simulink model "Model_6DOF"  (R2022b)
settings: Solver=VariableStepAuto  StartTime=0.0  StopTime=SimTime  RelTol=1e-6
InitFcn:
  | INIT_DATA
values from neighbouring files (symbols this model uses):
  g = 9.81    [aero_guid_dat.m]
  K_r = -0.02    [aero_guid_dat.m]
undefined symbols (not defined in the file or in its folder): a_L_c_max, a_N_c_max, b, C_bar, C_D_0, C_D_0_bar, C_D_alpha, C_D_d_e, C_L_0, C_L_0_bar, C_L_alpha, C_l_beta, C_l_d_a, C_L_d_e, C_l_d_r, C_l_p, C_L_q, C_l_r, C_m_0, C_m_alpha, C_m_d_e, C_m_q, C_n_beta, C_n_d_a, C_n_d_r, C_n_p, C_n_r, C_y_beta, C_y_d_a, C_y_d_r, C_y_p, C_y_r, d_T, da_max, da_rate_max, de_max, de_rate_max, dr_max, dr_rate_max, E, EA0, eR_0_IhI_Ih, eS_0_BE_Lh, eV_0_BE_Lh, G_cp, G_I, G_M, G_M_I, G_R, G_s, GC, I, INS_bias_f, INS_bias_omega, INS_imbalance_error, INS_scale_factor_error_f, INS_scale_factor_error_omega, k, K_beta, K_p ... (+34)
libraries: dspsrcs4 x11, matrix_library x6, simulink x5, sharedutil x3, aerolibasang x3, sharedtransform x2, simulink_extras x1, slpidlib x1
(part 1 of 2)
settings Model: Creator=Milad  LastModifiedBy=Mahdi
settings SolverCC: AlgebraicLoopSolver=TrustRegion
settings OptimizationCC: LifeSpan=inf
settings DebuggingCC: UnconnectedInputMsg=warning  UnconnectedOutputMsg=warning  UnconnectedLineMsg=warning  SFExecutionAtInitializationDiag=none  SFMachineParentedDataDiag=warning  ArithmeticOperatorsInVariantConditions=warning
settings HardwareCC: ProdBitPerSizeT=32  ProdBitPerPtrDiffT=32  ProdWordSize=32  ProdHWDeviceType=Specified
settings ModelReferenceCC: EnableRefExpFcnMdlSchedulingChecks=on
settings SFSimCC: CustomCodeUndefinedFunction=UseInterfaceOnly
settings CodeAppCC: StateflowObjectComments=on

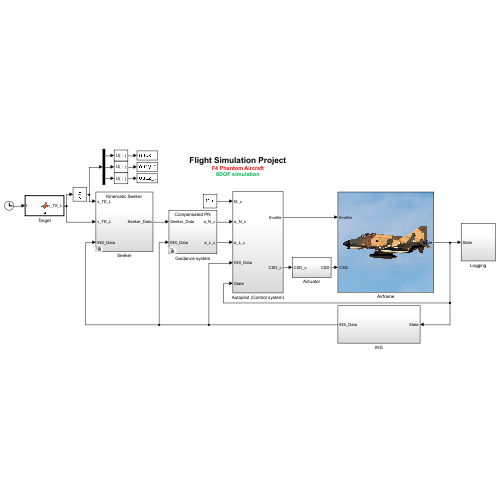
[thumbnail: Simulink's stored preview of the top-level diagram]
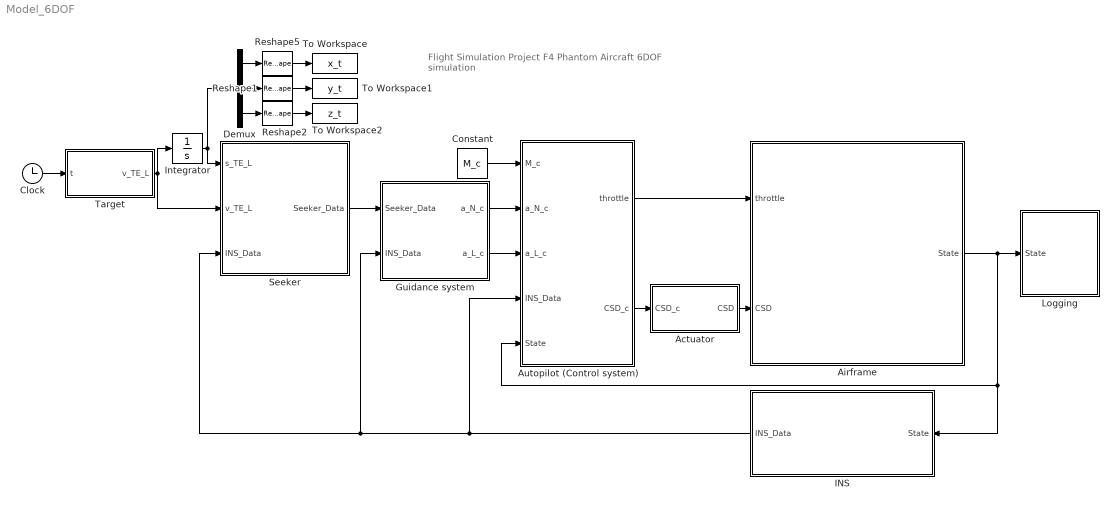
== system Model_6DOF ==
  note: Flight Simulation Project
      | F4 Phantom Aircraft
      | 6DOF simulation
  Actuator : Subsystem
  Airframe : Subsystem
      mask Display: image('E:\term courses\FS\project\phase1\70285_1544476732.jpg'); % Use "Edit Image" on toolstrip to change.
  Autopilot (Control system) : Subsystem
  Clock : Clock
  Constant : Constant  Value=M_c
  Demux : Demux  Outputs=3
  Guidance system : Subsystem  Variant=on  VariantControlMode=label  VariantControl=Choice  LabelModeActiveChoice=CPN
  INS : Subsystem
  Integrator : Integrator  InitialCondition=s_TE_L_0
  Logging : Subsystem
  Reshape1 : Reshape
  Reshape2 : Reshape
  Reshape5 : Reshape
  Seeker : Subsystem  Variant=on  VariantControlMode=label  VariantControl=Choice  LabelModeActiveChoice=kinematic
  Target : MATLAB Function  TreatAsAtomicUnit=on
  To Workspace : ToWorkspace  VariableName=x_t  SampleTime=out_SampleTime
  To Workspace1 : ToWorkspace  VariableName=y_t  SampleTime=out_SampleTime
  To Workspace2 : ToWorkspace  VariableName=z_t  SampleTime=out_SampleTime
  wires:
  Airframe/1(State) -> Logging/1(State), INS/1(State), Autopilot (Control system)/5(State)
  Autopilot (Control system)/1(throttle) -> Airframe/1(throttle)
  Autopilot (Control system)/2(CSD_c) -> Actuator/1(CSD_c)
  INS/1(INS_Data) -> Seeker/3(INS_Data), Guidance system/2(INS_Data), Autopilot (Control system)/4(INS_Data)
  Clock/1 -> Target/1(t)
  Reshape1/1 -> To Workspace1/1
  Reshape2/1 -> To Workspace2/1
  Demux/2 -> Reshape1/1
  Integrator/1 -> Demux/1, Seeker/1(s_TE_L)
  Target/1(v_TE_L) -> Seeker/2(v_TE_L), Integrator/1
  Demux/3 -> Reshape2/1
  Constant/1 -> Autopilot (Control system)/1(M_c)
  Demux/1 -> Reshape5/1
  Reshape5/1 -> To Workspace/1
  Actuator/1(CSD) -> Airframe/2(CSD)
  Guidance system/1(a_N_c) -> Autopilot (Control system)/2(a_N_c)
  Guidance system/2(a_L_c) -> Autopilot (Control system)/3(a_L_c)
  Seeker/1(Seeker_Data) -> Guidance system/1(Seeker_Data)

== system Model_6DOF/Actuator ==
  CSD_c : Inport
  Aileron Actuator Transfer Function : Subsystem
  Demux : Demux  Outputs=3
  Elevator Actuator Transfer Function : Subsystem
  Mux : Mux  Inputs=3
  Rudder Actuator Transfer Function : Subsystem
  CSD : Outport
  wires:
  Elevator Actuator Transfer Function/1(de) -> Mux/1
  Mux/1 -> CSD/1
  CSD_c/1 -> Demux/1
  Demux/1 -> Elevator Actuator Transfer Function/1(de_c)
  Demux/2 -> Aileron Actuator Transfer Function/1(da_c)
  Aileron Actuator Transfer Function/1(da) -> Mux/2
  Demux/3 -> Rudder Actuator Transfer Function/1(dr_c)
  Rudder Actuator Transfer Function/1(dr) -> Mux/3

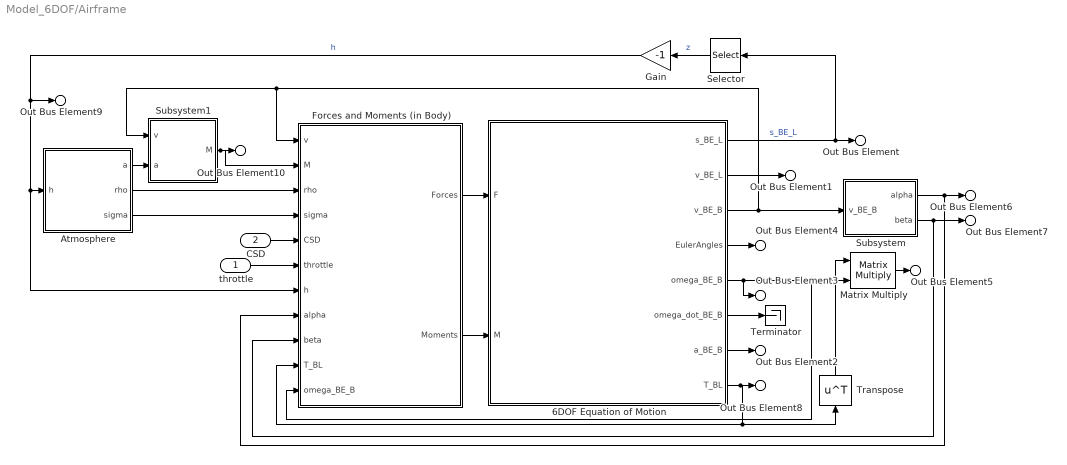
== system Model_6DOF/Airframe ==
  throttle : Inport
  CSD : Inport  Port=2
  6DOF Equation of Motion : Subsystem
  Atmosphere : MATLAB Function  TreatAsAtomicUnit=on
  Forces and Moments (in Body) : Subsystem
  Gain : Gain  Gain=-1
  Matrix Multiply : Product  Multiplication=Matrix(*)
  Selector : Selector  InputPortWidth=3  IndexOptions=Index vector (dialog)  Indices=3  OutputSizes=1
  Subsystem : Subsystem
  Subsystem1 : Subsystem
  Terminator : Terminator
  Transpose : Math  Operator=transpose
  Out Bus Element : Outport  PortName=State  Element=s_BE_L
  Out Bus Element1 : Outport  PortName=State  Element=v_BE_L
  Out Bus Element2 : Outport  PortName=State  Element=f_sp_B
  Out Bus Element3 : Outport  PortName=State  Element=omega_BE_B
  Out Bus Element4 : Outport  PortName=State  Element=EulerAngles
  Out Bus Element5 : Outport  PortName=State  Element=Omega_BE_L
  Out Bus Element6 : Outport  PortName=State  Element=alpha
  Out Bus Element7 : Outport  PortName=State  Element=beta
  Out Bus Element8 : Outport  PortName=State  Element=T_BL
  Out Bus Element9 : Outport  PortName=State  Element=h
  Out Bus Element10 : Outport  PortName=State  Element=M
  wires:
  6DOF Equation of Motion/2(v_BE_L) -> Out Bus Element1/1
  6DOF Equation of Motion/1(s_BE_L) -> Out Bus Element/1, Selector/1  "s_BE_L"
  Selector/1 -> Gain/1  "z"
  Gain/1 -> Out Bus Element9/1, Forces and Moments (in Body)/7(h), Atmosphere/1(h)  "h"
  Atmosphere/2(rho) -> Forces and Moments (in Body)/3(rho)
  Subsystem/1(alpha) -> Out Bus Element6/1, Forces and Moments (in Body)/8(alpha)
  Subsystem/2(beta) -> Out Bus Element7/1, Forces and Moments (in Body)/9(beta)
  throttle/1 -> Forces and Moments (in Body)/6(throttle)
  6DOF Equation of Motion/8(T_BL) -> Transpose/1, Forces and Moments (in Body)/10(T_BL), Out Bus Element8/1
  6DOF Equation of Motion/7(a_BE_B) -> Out Bus Element2/1
  Matrix Multiply/1 -> Out Bus Element5/1
  Atmosphere/3(sigma) -> Forces and Moments (in Body)/4(sigma)
  6DOF Equation of Motion/3(v_BE_B) -> Subsystem1/1(v), Forces and Moments (in Body)/1(v), Subsystem/1(v_BE_B)
  Forces and Moments (in Body)/1(Forces) -> 6DOF Equation of Motion/1(" F")
  Atmosphere/1(a) -> Subsystem1/2(a)
  Subsystem1/1(M) -> Forces and Moments (in Body)/2(M), Out Bus Element10/1
  Forces and Moments (in Body)/2(Moments) -> 6DOF Equation of Motion/2(M)
  CSD/1 -> Forces and Moments (in Body)/5(CSD)
  6DOF Equation of Motion/4(EulerAngles) -> Out Bus Element4/1
  6DOF Equation of Motion/5(omega_BE_B) -> Out Bus Element3/1, Matrix Multiply/2, Forces and Moments (in Body)/11(omega_BE_B)
  Transpose/1 -> Matrix Multiply/1
  6DOF Equation of Motion/6(omega_dot_BE_B) -> Terminator/1

== system Model_6DOF/Autopilot (Control system) ==
  M_c : Inport
  a_N_c : Inport  Port=2
  a_L_c : Inport  Port=3
  INS_Data : Inport  Port=4
  BusElementIn : Inport  Port=5  PortName=State  Element=h
  BusElementIn1 : Inport  Port=5  PortName=State  Element=beta
  BusElementIn2 : Inport  Port=5  PortName=State  Element=alpha
  BusElementIn3 : Inport  Port=5  PortName=State  Element=M
  Acceleration Autopilot : Subsystem
  Mach Hold Autopilot : Subsystem
  Mux : Mux  Inputs=3
  beta control : Subsystem
  throttle : Outport
  CSD_c : Outport  Port=2
  wires:
  M_c/1 -> Mach Hold Autopilot/1(M_c)
  Mach Hold Autopilot/1(throttle) -> throttle/1
  Acceleration Autopilot/1(de_c) -> Mux/1  "de_c"
  a_N_c/1 -> Acceleration Autopilot/1(a_N_c)
  a_L_c/1 -> Acceleration Autopilot/2(a_L_c)
  INS_Data/1 -> beta control/1(INS_Data), Acceleration Autopilot/3(INS_Data)
  Acceleration Autopilot/2(da_c) -> Mux/2  "da_c"
  beta control/1(dr_c) -> Mux/3
  Mux/1 -> CSD_c/1
  BusElementIn1/1 -> beta control/2(beta)
  BusElementIn/1 -> Mach Hold Autopilot/3(h)
  BusElementIn2/1 -> Mach Hold Autopilot/4(alpha)
  BusElementIn3/1 -> Mach Hold Autopilot/2(M)

== system Model_6DOF/Guidance system ==
  Seeker_Data : Inport
  INS_Data : Inport  Port=2
  Compensated PN : Subsystem  VariantControl=CPN
  IPN : Subsystem  VariantControl=IPN
  Optimal Guidance : Subsystem  VariantControl=OG
  a_N_c : Outport
  a_L_c : Outport  Port=2

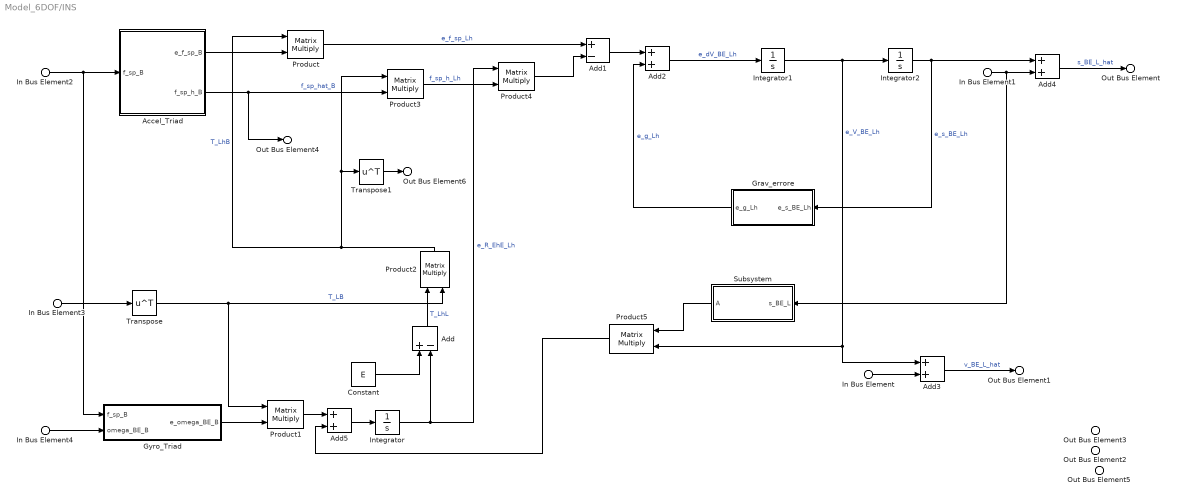
== system Model_6DOF/INS ==
  In Bus Element : Inport  PortName=State  Element=v_BE_L
  In Bus Element1 : Inport  PortName=State  Element=s_BE_L
  In Bus Element2 : Inport  PortName=State  Element=f_sp_B
  In Bus Element3 : Inport  PortName=State  Element=T_BL
  In Bus Element4 : Inport  PortName=State  Element=omega_BE_B
  Accel_Triad : Subsystem
  Add : Sum  Inputs=+-
  Add1 : Sum  Inputs=+-
  Add{2..5} (4 alike) : Sum
  Constant : Constant  Value=E
  Grav_errore : Subsystem
  Gyro_Triad : Subsystem
  Integrator : Integrator  InitialCondition=eR_0_IhI_Ih
  Integrator1 : Integrator  InitialCondition=eV_0_BE_Lh
  Integrator2 : Integrator  InitialCondition=eS_0_BE_Lh
  Product{,1..5} (6 alike) : Product  Multiplication=Matrix(*)
  Subsystem : Subsystem
  Transpose : Math  Operator=transpose
  Transpose1 : Math  Operator=transpose
  Out Bus Element : Outport  PortName=INS_Data  Element=s_BE_L_hat
  Out Bus Element1 : Outport  PortName=INS_Data  Element=v_BE_L_hat
  Out Bus Element2 : Outport  PortName=INS_Data  Element=phi_theta_psi
  Out Bus Element3 : Outport  PortName=INS_Data  Element=pqr
  Out Bus Element4 : Outport  PortName=INS_Data  Element=f_sp_hat_B
  Out Bus Element5 : Outport  PortName=INS_Data  Element=a_m
  Out Bus Element6 : Outport  PortName=INS_Data  Element=T_BL_hat
  wires:
  ? -> Out Bus Element3/1
  ? -> Out Bus Element2/1
  Accel_Triad/2(f_sp_h_B) -> Out Bus Element4/1, Product3/2  "f_sp_hat_B"
  Transpose1/1 -> Out Bus Element6/1
  ? -> Out Bus Element5/1
  In Bus Element/1 -> Add3/2
  Product5/1 -> Add5/2
  Product1/1 -> Add5/1
  Integrator2/1 -> Grav_errore/1(e_s_BE_Lh), Add4/1  "e_s_BE_Lh"
  Integrator1/1 -> Integrator2/1, Product5/2, Add3/1  "e_V_BE_Lh"
  Accel_Triad/1(e_f_sp_B) -> Product/2
  Product3/1 -> Product4/2  "f_sp_h_Lh"
  Gyro_Triad/1(e_omega_BE_B) -> Product1/2
  Add/1 -> Product2/1  "T_LhL"
  Add5/1 -> Integrator/1
  Product/1 -> Add1/1  "e_f_sp_Lh"
  Add2/1 -> Integrator1/1  "e_dV_BE_Lh"
  Constant/1 -> Add/1
  Add4/1 -> Out Bus Element/1  "s_BE_L_hat"
  Add3/1 -> Out Bus Element1/1  "v_BE_L_hat"
  Integrator/1 -> Add/2, Product4/1  "e_R_EhE_Lh"
  Product4/1 -> Add1/2
  Add1/1 -> Add2/1
  Product2/1 -> Product3/1, Transpose1/1, Product/1  "T_LhB"
  Grav_errore/1(e_g_Lh) -> Add2/2  "e_g_Lh"
  Transpose/1 -> Product1/1, Product2/2  "T_LB"
  Subsystem/1(A) -> Product5/1
  In Bus Element1/1 -> Subsystem/1(s_BE_L), Add4/2
  In Bus Element2/1 -> Gyro_Triad/1(f_sp_B), Accel_Triad/1(f_sp_B)
  In Bus Element3/1 -> Transpose/1
  In Bus Element4/1 -> Gyro_Triad/2(omega_BE_B)

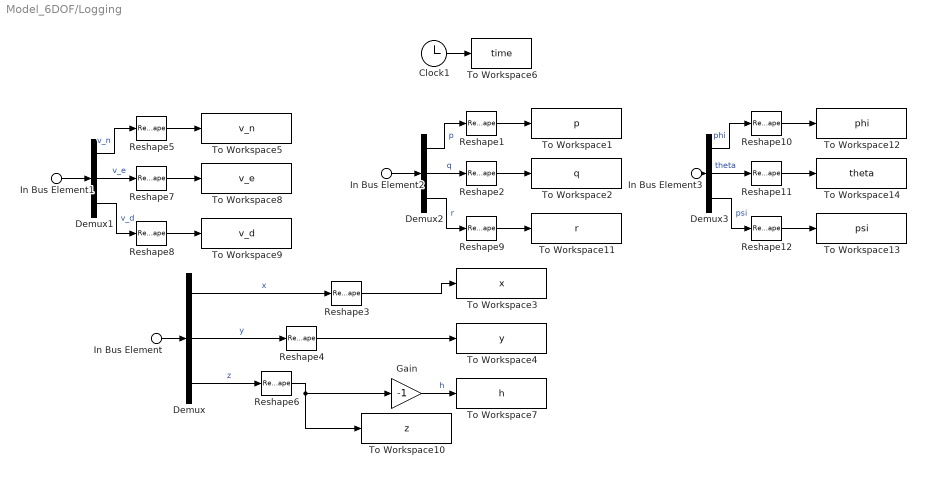
== system Model_6DOF/Logging ==
  In Bus Element : Inport  PortName=State  Element=s_BE_L
  In Bus Element1 : Inport  PortName=State  Element=v_BE_L
  In Bus Element2 : Inport  PortName=State  Element=omega_BE_B
  In Bus Element3 : Inport  PortName=State  Element=EulerAngles
  Clock1 : Clock
  Demux{,1..3} (4 alike) : Demux  Outputs=3
  Gain : Gain  Gain=-1
  Reshape{1..12} (12 alike) : Reshape
  To Workspace1 : ToWorkspace  VariableName=p  SampleTime=out_SampleTime
  To Workspace10 : ToWorkspace  VariableName=z  SampleTime=out_SampleTime
  To Workspace11 : ToWorkspace  VariableName=r  SampleTime=out_SampleTime
  To Workspace12 : ToWorkspace  VariableName=phi  SampleTime=out_SampleTime
  To Workspace13 : ToWorkspace  VariableName=psi  SampleTime=out_SampleTime
  To Workspace14 : ToWorkspace  VariableName=theta  SampleTime=out_SampleTime
  To Workspace2 : ToWorkspace  VariableName=q  SampleTime=out_SampleTime
  To Workspace3 : ToWorkspace  VariableName=x  SampleTime=out_SampleTime
  To Workspace4 : ToWorkspace  VariableName=y  SampleTime=out_SampleTime
  To Workspace5 : ToWorkspace  VariableName=v_n  SampleTime=out_SampleTime
  To Workspace6 : ToWorkspace  VariableName=time  SampleTime=out_SampleTime
  To Workspace7 : ToWorkspace  VariableName=h  SampleTime=out_SampleTime
  To Workspace8 : ToWorkspace  VariableName=v_e  SampleTime=out_SampleTime
  To Workspace9 : ToWorkspace  VariableName=v_d  SampleTime=out_SampleTime
  wires:
  Clock1/1 -> To Workspace6/1
  Demux/3 -> Reshape6/1  "z"
  Demux/1 -> Reshape3/1  "x"
  Gain/1 -> To Workspace7/1  "h"
  Demux/2 -> Reshape4/1  "y"
  In Bus Element1/1 -> Demux1/1
  Demux1/1 -> Reshape5/1  "v_n"
  Demux1/2 -> Reshape7/1  "v_e"
  Demux1/3 -> Reshape8/1  "v_d"
  Reshape3/1 -> To Workspace3/1
  Reshape4/1 -> To Workspace4/1
  Reshape6/1 -> Gain/1, To Workspace10/1
  Reshape5/1 -> To Workspace5/1
  Reshape7/1 -> To Workspace8/1
  Reshape8/1 -> To Workspace9/1
  In Bus Element/1 -> Demux/1
  In Bus Element2/1 -> Demux2/1
  Demux2/3 -> Reshape9/1  "r"
  Reshape9/1 -> To Workspace11/1
  Reshape2/1 -> To Workspace2/1
  Demux2/2 -> Reshape2/1  "q"
  Demux2/1 -> Reshape1/1  "p"
  Reshape1/1 -> To Workspace1/1
  Reshape10/1 -> To Workspace12/1
  Demux3/1 -> Reshape10/1  "phi"
  Demux3/2 -> Reshape11/1  "theta"
  Reshape11/1 -> To Workspace14/1
  Demux3/3 -> Reshape12/1  "psi"
  In Bus Element3/1 -> Demux3/1
  Reshape12/1 -> To Workspace13/1

== system Model_6DOF/Seeker ==
  s_TE_L : Inport
  v_TE_L : Inport  Port=2
  INS_Data : Inport  Port=3
  Dynamic Seeker : Subsystem  VariantControl=dynamic
  Kinematic Seeker : Subsystem  VariantControl=kinematic
  Seeker_Data : Outport

== system Model_6DOF/Actuator/Aileron Actuator Transfer Function ==
  da_c : Inport
  Gain : Gain  Gain=omega_n_da^2
  Gain1 : Gain  Gain=2*zeta_da
  Gain2 : Gain  Gain=omega_n_da
  Integrator : Integrator
  Integrator1 : Integrator
  Rate Saturation : Saturate  UpperLimit=da_rate_max  LowerLimit=-da_rate_max
  Sum : Sum  Inputs=|+-
  Sum1 : Sum  Inputs=|+-
  deflection saturation : Saturate  UpperLimit=da_max  LowerLimit=-da_max
  da : Outport
  wires:
  deflection saturation/1 -> da/1, Sum/2
  Integrator1/1 -> deflection saturation/1
  Rate Saturation/1 -> Gain1/1, Integrator1/1
  Integrator/1 -> Rate Saturation/1
  Sum1/1 -> Integrator/1
  Gain2/1 -> Sum1/2
  Gain1/1 -> Gain2/1
  Gain/1 -> Sum1/1
  Sum/1 -> Gain/1
  da_c/1 -> Sum/1

== system Model_6DOF/Actuator/Elevator Actuator Transfer Function ==
  de_c : Inport
  Gain : Gain  Gain=omega_n_de^2
  Gain1 : Gain  Gain=2*zeta_de
  Gain2 : Gain  Gain=omega_n_de
  Integrator : Integrator
  Integrator1 : Integrator
  Rate Saturation : Saturate  UpperLimit=de_rate_max  LowerLimit=-de_rate_max
  Sum : Sum  Inputs=|+-
  Sum1 : Sum  Inputs=|+-
  deflection saturation : Saturate  UpperLimit=de_max  LowerLimit=-de_max
  de : Outport
  wires:
  de_c/1 -> Sum/1
  Sum/1 -> Gain/1
  Gain/1 -> Sum1/1
  Gain1/1 -> Gain2/1
  Gain2/1 -> Sum1/2
  Sum1/1 -> Integrator/1
  Integrator/1 -> Rate Saturation/1
  Rate Saturation/1 -> Integrator1/1, Gain1/1
  Integrator1/1 -> deflection saturation/1
  deflection saturation/1 -> Sum/2, de/1

== system Model_6DOF/Actuator/Rudder Actuator Transfer Function ==
  dr_c : Inport
  Gain : Gain  Gain=omega_n_dr^2
  Gain1 : Gain  Gain=2*zeta_dr
  Gain2 : Gain  Gain=omega_n_dr
  Integrator : Integrator
  Integrator1 : Integrator
  Rate Saturation : Saturate  UpperLimit=dr_rate_max  LowerLimit=-dr_rate_max
  Sum : Sum  Inputs=|+-
  Sum1 : Sum  Inputs=|+-
  deflection saturation : Saturate  UpperLimit=dr_max  LowerLimit=-dr_max
  dr : Outport
  wires:
  dr_c/1 -> Sum/1
  Sum/1 -> Gain/1
  Gain/1 -> Sum1/1
  Gain1/1 -> Gain2/1
  Gain2/1 -> Sum1/2
  Sum1/1 -> Integrator/1
  Integrator/1 -> Rate Saturation/1
  Rate Saturation/1 -> Integrator1/1, Gain1/1
  Integrator1/1 -> deflection saturation/1
  deflection saturation/1 -> Sum/2, dr/1

== system Model_6DOF/Airframe/6DOF Equation of Motion ==
  " F" : Inport
  M : Inport  Port=2
  Demux : Demux  Outputs=3
  Integrator : Integrator  InitialCondition=Vb0
  Integrator1 : Integrator  InitialCondition=X0
  Integrator2 : Integrator  InitialCondition=RR0
  Integrator3 : Integrator  InitialCondition=EA0  WrapState=on
  Mux : Mux  Inputs=3
  Rotation Angles to Direction Cosine Matrix : sharedtransform/Rotation Angles to Direction Cosine Matrix  rotationOrder=ZYX  aMode=aMode
  Rotational Dynamics (kinetics) : Subsystem
  Rotational Kinematics : Subsystem
  Saturation : Saturate  UpperLimit=0  LowerLimit=-inf
  Selector : Selector  InputPortWidth=3  IndexOptions=Index vector (dialog)  Indices=[3 2 1]  OutputSizes=1
  Transitional Dynamics (kinetics) : Subsystem
  "Transitional Kinematics " : Subsystem
  s_BE_L : Outport
  v_BE_L : Outport  Port=2
  v_BE_B : Outport  Port=3
  EulerAngles : Outport  Port=4
  omega_BE_B : Outport  Port=5
  omega_dot_BE_B : Outport  Port=6
  a_BE_B : Outport  Port=7
  T_BL : Outport  Port=8
  wires:
  Rotational Kinematics/1(Euler Rates) -> Integrator3/1  "phidot,thetadot,psidot"
  M/1 -> Rotational Dynamics (kinetics)/1(Moment)
  Demux/1 -> Mux/1
  " F"/1 -> Transitional Dynamics (kinetics)/1(" F")
  Saturation/1 -> Mux/3
  Integrator1/1 -> Demux/1
  Demux/2 -> Mux/2
  Integrator2/1 -> Transitional Dynamics (kinetics)/2(p,q,r), Rotational Kinematics/2(omega_body), Rotational Dynamics (kinetics)/2(p,q,r), omega_BE_B/1  "omega_body"
  Rotational Dynamics (kinetics)/1(omegadot_body) -> omega_dot_BE_B/1, Integrator2/1  "pdot,qdot,rdot"
  "Transitional Kinematics "/1(V_earth) -> v_BE_L/1, Integrator1/1  "xdot,ydot,zdot"
  Transitional Dynamics (kinetics)/1(Vdot_body) -> Integrator/1  "udot,vdot,wdot"
  Mux/1 -> s_BE_L/1  "Positiopn"
  Demux/3 -> Saturation/1
  Integrator3/1 -> "Transitional Kinematics "/2(Euler Angles), Selector/1, Rotational Kinematics/1(Euler Angles), EulerAngles/1
  Integrator/1 -> v_BE_B/1, Transitional Dynamics (kinetics)/3(V_body), "Transitional Kinematics "/1(V_body)  "V_body"
  Selector/1 -> Rotation Angles to Direction Cosine Matrix/1
  Rotation Angles to Direction Cosine Matrix/1 -> T_BL/1
  Transitional Dynamics (kinetics)/2(a_BE_B) -> a_BE_B/1

== system Model_6DOF/Airframe/Forces and Moments (in Body) ==
  v : Inport
  M : Inport  Port=2
  rho : Inport  Port=3
  sigma : Inport  Port=4
  CSD : Inport  Port=5
  throttle : Inport  Port=6
  h : Inport  Port=7
  alpha : Inport  Port=8
  beta : Inport  Port=9
  T_BL : Inport  Port=10
  omega_BE_B : Inport  Port=11
  Aerodynamics Forces & Moments : Subsystem
  Gain : Gain  Gain=m
  Gravitational Acceleration : Subsystem
  Propulsion : Subsystem
  Sum1 : Sum  Inputs=2
  Sum2 : Sum  Inputs=3
  Terminator : Terminator
  Forces : Outport
  Moments : Outport  Port=2
  wires:
  alpha/1 -> Aerodynamics Forces & Moments/2(alpha)
  rho/1 -> Aerodynamics Forces & Moments/5(rho)
  beta/1 -> Aerodynamics Forces & Moments/3(beta)
  throttle/1 -> Propulsion/2(throttle)
  v/1 -> Aerodynamics Forces & Moments/1(v)
  M/1 -> Terminator/1
  sigma/1 -> Propulsion/3(sigma)
  h/1 -> Propulsion/1(h)
  Gravitational Acceleration/1(g) -> Gain/1  "Gravitational Acceleration"
  Sum1/1 -> Moments/1
  Propulsion/2(F_T_B) -> Sum2/2  "Thrust Forces"
  Propulsion/1(M_T_B) -> Sum1/2  "Thrust Moments"
  Sum2/1 -> Forces/1
  Aerodynamics Forces & Moments/1(F_A_B) -> Sum2/1  "Aerodynamic Forces"
  Gain/1 -> Sum2/3
  Aerodynamics Forces & Moments/2(M_A_B) -> Sum1/1  "Aerodynamics Moments"
  T_BL/1 -> Gravitational Acceleration/1(T_BL)
  CSD/1 -> Aerodynamics Forces & Moments/4(CSD)
  omega_BE_B/1 -> Aerodynamics Forces & Moments/6(omega_BE_B)

== system Model_6DOF/Airframe/Subsystem ==
  note: beta = arcsin (v1/VP1)
  note: alpha = arctan (w1/u1)
  v_BE_B : Inport
  Atan2 : Trigonometry  Operator=atan2
  Divide : Product  Inputs=*/
  Pow : Math  Operator=magnitude^2  RndMeth=Zero
  Scope : Scope
  Selector : Selector  InputPortWidth=3  IndexOptions=Index vector (dialog)  Indices=[2]  OutputSizes=1
  Selector1 : Selector  InputPortWidth=3  IndexOptions=Index vector (dialog)  Indices=[3]  OutputSizes=1
  Selector2 : Selector  InputPortWidth=3  IndexOptions=Index vector (dialog)  Indices=[1]  OutputSizes=1
  Sqrt : Sqrt
  Sum of Elements : Sum  Inputs=+
  To Workspace : ToWorkspace  VariableName=alpha  SaveFormat=Timeseries  SampleTime=-1
  To Workspace1 : ToWorkspace  VariableName=beta  SaveFormat=Timeseries  SampleTime=-1
  Trigonometric Function : Trigonometry  Operator=asin
  alpha : Outport
  beta : Outport  Port=2
  wires:
  Sum of Elements/1 -> Sqrt/1
  Pow/1 -> Sum of Elements/1
  Trigonometric Function/1 -> To Workspace1/1, beta/1
  Divide/1 -> Trigonometric Function/1
  Sqrt/1 -> Divide/2
  Selector/1 -> Divide/1  "v"
  v_BE_B/1 -> Selector2/1, Selector1/1, Pow/1, Selector/1  "V"
  Selector2/1 -> Atan2/2  "u"
  Selector1/1 -> Atan2/1  "w"
  Atan2/1 -> Scope/1, alpha/1, To Workspace/1

== system Model_6DOF/Airframe/Subsystem1 ==
  v : Inport
  a : Inport  Port=2
  Divide : Product  Inputs=*/
  Square : Math  Operator=square
  Square1 : Math  Operator=square
  Sum of Elements : Sum  Inputs=+
  M : Outport  PortDimensions=1
  wires:
  Divide/1 -> M/1
  a/1 -> Divide/2
  v/1 -> Square/1
  Square/1 -> Sum of Elements/1
  Sum of Elements/1 -> Square1/1
  Square1/1 -> Divide/1

== system Model_6DOF/Autopilot (Control system)/Acceleration Autopilot ==
  a_N_c : Inport
  a_L_c : Inport  Port=2
  In Bus Element1 : Inport  Port=3  PortName=INS_Data
  In Bus Element : Inport  Port=3  PortName=INS_Data  Element=phi_theta_psi
  Acceleration Autopilot : Subsystem
  Cos : Trigonometry  Operator=cos
  Product : Product  Inputs=*/
  Selector : Selector  InputPortWidth=3  IndexOptions=Index vector (dialog)  Indices=1  OutputSizes=1
  phi controller : Subsystem
  de_c : Outport
  da_c : Outport  Port=2
  wires:
  a_N_c/1 -> Product/1
  Cos/1 -> Product/2
  Product/1 -> Acceleration Autopilot/1(a_N_c)  "a_N_c_BTT"
  In Bus Element1/1 -> phi controller/1(INS_Data), Acceleration Autopilot/2(INS_Data)
  a_L_c/1 -> phi controller/2(a_L_c)
  Acceleration Autopilot/1(d_e_c) -> de_c/1  "d_e_c"
  In Bus Element/1 -> Selector/1
  Selector/1 -> Cos/1  "phi"
  phi controller/1(d_a_c) -> da_c/1

== system Model_6DOF/Autopilot (Control system)/Mach Hold Autopilot ==
  M_c : Inport
  M : Inport  Port=2  PortDimensions=1
  h : Inport  Port=3  PortDimensions=1
  alpha : Inport  Port=4  PortDimensions=1
  Add : Sum  Inputs=+-
  Add1 : Sum
  PID Controller : slpidlib/PID Controller  Controller=PI  Form=Parallel  TimeDomain=Continuous-time  UseExternalTs=off  SampleTime=-1  IntegratorMethod=Forward Euler  FilterMethod=Forward Euler  ControllerParametersSource=internal  P=G_M  I=G_M_I  UseKiTs=off  D=179.966531165973  N=386.734790036957  UseFilter=on  TunerSelectOption=Transfer Function Based (PID Tuner App)  InitialConditionSource=internal  InitialConditionForIntegrator=0  InitialConditionForFilter=0  DifferentiatorICPrevScaledInput=0  ExternalReset=none  TrackingMode=off  Kt=1  LimitOutput=on  SatLimitsSource=internal  UpperSaturationLimit=1  LowerSaturationLimit=-1  LinearizeAsGain=on  AntiWindupMode=clamping  Kb=1  LimitIntegrator=off  UpperIntegratorSaturationLimit=inf  LowerIntegratorSaturationLimit=-inf  POutMin=[]  POutMax=[]  IOutMin=[]  IOutMax=[]  DOutMin=[]  DOutMax=[]  NOutMin=[]  NOutMax=[]  SumOutMin=[]  SumOutMax=[]  SaturationOutMin=[]  SaturationOutMax=[]  PParamMin=[]  PParamMax=[]  IParamMin=[]  IParamMax=[]  DParamMin=[]  DParamMax=[]  NParamMin=[]  NParamMax=[]  KbParamMin=[]  KbParamMax=[]  KtParamMin=[]  KtParamMax=[]  KbOutMin=[]  KbOutMax=[]  KtOutMin=[]  KtOutMax=[]  IntegratorOutMin=[]  IntegratorOutMax=[]  FilterOutMin=[]  FilterOutMax=[]  SumI1OutMin=[]  SumI1OutMax=[]  SumI2OutMin=[]  SumI2OutMax=[]  SumI3OutMin=[]  SumI3OutMax=[]  SumI4OutMin=[]  SumI4OutMax=[]  SumDOutMin=[]  SumDOutMax=[]  DifferentiatorOutMin=[]  DifferentiatorOutMax=[]  FilterDiffOutCoefMin=[]  FilterDiffOutCoefMax=[]  ReciprocalOutMin=[]  ReciprocalOutMax=[]  SumDenOutMin=[]  SumDenOutMax=[]  SumNumOutMin=[]  SumNumOutMax=[]  DivideOutMin=[]  DivideOutMax=[]  UdiffTsProdOutMin=[]  UdiffTsProdOutMax=[]  NTsProdOutMin=[]  NTsProdOutMax=[]  UintegralTsProdOutMin=[]  UintegralTsProdOutMax=[]  UngainTsProdOutMin=[]  UngainTsProdOutMax=[]  ClampingZeroOutDataTypeStr=Inherit: Inherit via back propagation  ClampingZeroOutMin=[]  ClampingZeroOutMax=[]  FilterDenConstantOutDataTypeStr=Inherit: Inherit via back propagation  FilterDenConstantOutMin=[]  FilterDenConstantOutMax=[]  PCopyOutDataTypeStr=Inherit: Inherit via back propagation  PCopyOutMin=[]  PCopyOutMax=[]  NCopyOutDataTypeStr=Inherit: Inherit via back propagation  NCopyOutMin=[]  NCopyOutMax=[]  IntegratorContinuousStateAttributes=''  IntegratorStateMustResolveToSignalObject=off  IntegratorRTWStateStorageClass=Auto  FilterContinuousStateAttributes=''  FilterStateMustResolveToSignalObject=off  FilterRTWStateStorageClass=Auto  ParallelPVariant=InternalParameters  IdealPVariant=Disabled  IVariant=InternalParameters  DVariant=Disabled  IntegratorVariant=Continuous  SatVariant=Enabled  AWVariant=ContClampingParallel  PCopyVariant=Disabled  TRVariant=Disabled  FdbkBlocksVariant=Forward  IdealPFdbkVariant=Disabled  SatFdbkVariant=Disabled  DerivativeFilterVariant=Disabled  NVariant=Disabled  NCopyVariant=Disabled_SignalSpec  FilterICVariant=Disabled  IntegratorICVariant=InternalICs  ExternalResetVariant=Disabled  TRSumVariant=Passthrough  SumFdbkVariant=Disabled  SumVariant=Sum_PI  TsampFilterVariant=InternalTs  TsampNgainVariant=Passthrough  TsampIntegralVariant=Passthrough  ExternalSaturationOutDataTypeStr=Inherit: Same as second input
  Saturation : Saturate  UpperLimit=1  LowerLimit=0
  Scope : Scope
  Scope1 : Scope
  Scope2 : Scope
  throttle required : Subsystem
  throttle : Outport  PortDimensions=1
  wires:
  Saturation/1 -> Scope2/1, throttle/1
  M_c/1 -> Add/1, throttle required/3(M_c)
  h/1 -> throttle required/1(h)
  alpha/1 -> throttle required/2(alpha)
  M/1 -> Add/2
  throttle required/1(throttle_req) -> Scope/1, Add1/1
  Add1/1 -> Scope1/1, Saturation/1
  PID Controller/1 -> Add1/2
  Add/1 -> PID Controller/1

== system Model_6DOF/Autopilot (Control system)/beta control ==
  In Bus Element : Inport  PortName=INS_Data  Element=pqr
  beta : Inport  Port=2
  Add : Sum  Inputs=-+
  Gain : Gain  Gain=K_beta
  Gain1 : Gain  Gain=K_r
  Gain2 : Gain  Gain=-1
  Saturation : Saturate  UpperLimit=r_c_max  LowerLimit=-r_c_max
  Saturation1 : Saturate  UpperLimit=dr_max  LowerLimit=-dr_max
  Selector : Selector  InputPortWidth=3  IndexOptions=Index vector (dialog)  Indices=3  OutputSizes=1
  dr_c : Outport
  wires:
  beta/1 -> Gain/1
  Saturation/1 -> Add/2  "r_c"
  Gain/1 -> Saturation/1
  In Bus Element/1 -> Selector/1
  Selector/1 -> Add/1
  Add/1 -> Gain1/1
  Gain1/1 -> Saturation1/1
  Saturation1/1 -> Gain2/1
  Gain2/1 -> dr_c/1

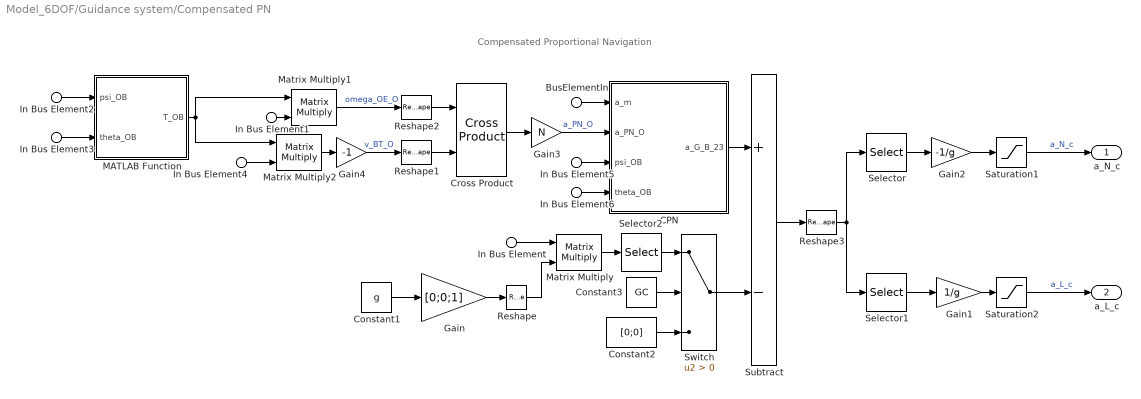
== system Model_6DOF/Guidance system/Compensated PN ==
  note: Compensated Proportional Navigation
  In Bus Element1 : Inport  PortName=Seeker_Data  Element=omega_OE_B
  In Bus Element2 : Inport  PortName=Seeker_Data  Element=psi_SB
  In Bus Element5 : Inport  PortName=Seeker_Data  Element=psi_SB
  In Bus Element3 : Inport  PortName=Seeker_Data  Element=theta_SB
  In Bus Element6 : Inport  PortName=Seeker_Data  Element=theta_SB
  In Bus Element4 : Inport  PortName=Seeker_Data  Element=v_TB_B
  In Bus Element : Inport  Port=2  PortName=INS_Data  Element=T_BL
  BusElementIn : Inport  Port=2  PortName=INS_Data  Element=a_m
  CPN : MATLAB Function  TreatAsAtomicUnit=on
  Constant1 : Constant  Value=g
  Constant2 : Constant  Value=[0;0]
  Constant3 : Constant  Value=GC
  Cross Product : matrix_library/Cross Product
  Gain : Gain  Gain=[0;0;1]
  Gain1 : Gain  Gain=1/g
  Gain2 : Gain  Gain=-1/g
  Gain3 : Gain  Gain=N
  Gain4 : Gain  Gain=-1
  MATLAB Function : MATLAB Function  TreatAsAtomicUnit=on
  Matrix Multiply : Product  Multiplication=Matrix(*)
  Matrix Multiply1 : Product  Multiplication=Matrix(*)
  Matrix Multiply2 : Product  Multiplication=Matrix(*)
  Reshape : Reshape  OutputDimensionality=Column vector (2-D)
  Reshape1 : Reshape  OutputDimensionality=Column vector (2-D)
  Reshape2 : Reshape  OutputDimensionality=Column vector (2-D)
  Reshape3 : Reshape
  Saturation1 : Saturate  UpperLimit=a_N_c_max  LowerLimit=-a_N_c_max
  Saturation2 : Saturate  UpperLimit=a_L_c_max  LowerLimit=-a_L_c_max
  Selector : Selector  InputPortWidth=2  IndexOptions=Index vector (dialog)  Indices=2  OutputSizes=1
  Selector1 : Selector  InputPortWidth=2  IndexOptions=Index vector (dialog)  Indices=1  OutputSizes=1
  Selector2 : Selector  InputPortWidth=3  IndexOptions=Index vector (dialog)  Indices=[2 3]  OutputSizes=1
  Subtract : Sum  Inputs=+-
  Switch : Switch  Criteria=u2 > Threshold  SaturateOnIntegerOverflow=off  InputSameDT=off
  a_N_c : Outport
  a_L_c : Outport  Port=2
  wires:
  In Bus Element/1 -> Matrix Multiply/1
  Gain4/1 -> Reshape1/1  "v_BT_O"
  Gain1/1 -> Saturation2/1
  Gain2/1 -> Saturation1/1
  Constant2/1 -> Switch/3
  Constant3/1 -> Switch/2
  Matrix Multiply/1 -> Selector2/1
  Switch/1 -> Subtract/2
  Reshape3/1 -> Selector1/1, Selector/1
  Saturation2/1 -> a_L_c/1  "a_L_c"
  Saturation1/1 -> a_N_c/1  "a_N_c"
  Reshape2/1 -> Cross Product/1
  Reshape1/1 -> Cross Product/2
  Selector1/1 -> Gain1/1
  Selector/1 -> Gain2/1
  Reshape/1 -> Matrix Multiply/2
  Gain/1 -> Reshape/1
  Constant1/1 -> Gain/1
  Cross Product/1 -> Gain3/1
  In Bus Element2/1 -> MATLAB Function/1(psi_OB)
  In Bus Element3/1 -> MATLAB Function/2(theta_OB)
  Gain3/1 -> CPN/2(a_PN_O)  "a_PN_O"
  MATLAB Function/1(T_OB) -> Matrix Multiply1/1, Matrix Multiply2/1
  BusElementIn/1 -> CPN/1(a_m)
  Subtract/1 -> Reshape3/1
  Matrix Multiply1/1 -> Reshape2/1  "omega_OE_O"
  In Bus Element1/1 -> Matrix Multiply1/2
  In Bus Element4/1 -> Matrix Multiply2/2
  Matrix Multiply2/1 -> Gain4/1
  Selector2/1 -> Switch/1
  In Bus Element5/1 -> CPN/3(psi_OB)
  In Bus Element6/1 -> CPN/4(theta_OB)
  CPN/1(a_G_B_23) -> Subtract/1

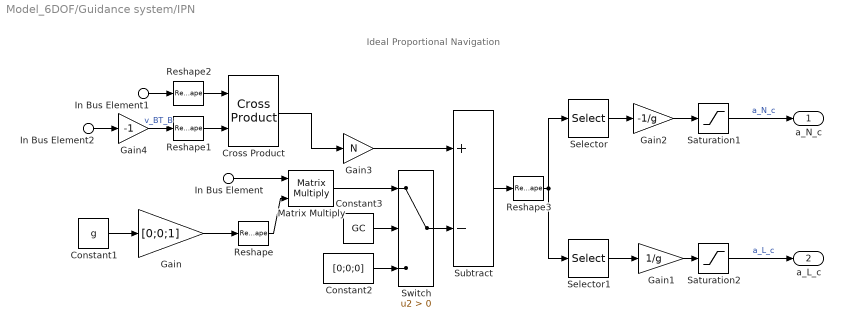
== system Model_6DOF/Guidance system/IPN ==
  note: Ideal Proportional Navigation
  In Bus Element1 : Inport  PortName=Seeker_Data  Element=omega_OE_B
  In Bus Element2 : Inport  PortName=Seeker_Data  Element=v_TB_B
  In Bus Element : Inport  Port=2  PortName=INS_Data  Element=T_BL
  Constant1 : Constant  Value=g
  Constant2 : Constant  Value=[0;0;0]
  Constant3 : Constant  Value=GC
  Cross Product : matrix_library/Cross Product
  Gain : Gain  Gain=[0;0;1]
  Gain1 : Gain  Gain=1/g
  Gain2 : Gain  Gain=-1/g
  Gain3 : Gain  Gain=N
  Gain4 : Gain  Gain=-1
  Matrix Multiply : Product  Multiplication=Matrix(*)
  Reshape : Reshape  OutputDimensionality=Column vector (2-D)
  Reshape1 : Reshape  OutputDimensionality=Column vector (2-D)
  Reshape2 : Reshape  OutputDimensionality=Column vector (2-D)
  Reshape3 : Reshape
  Saturation1 : Saturate  UpperLimit=a_N_c_max  LowerLimit=-a_N_c_max
  Saturation2 : Saturate  UpperLimit=a_L_c_max  LowerLimit=-a_L_c_max
  Selector : Selector  InputPortWidth=3  IndexOptions=Index vector (dialog)  Indices=3  OutputSizes=1
  Selector1 : Selector  InputPortWidth=3  IndexOptions=Index vector (dialog)  Indices=2  OutputSizes=1
  Subtract : Sum  Inputs=+-
  Switch : Switch  Criteria=u2 > Threshold  SaturateOnIntegerOverflow=off  InputSameDT=off
  a_N_c : Outport
  a_L_c : Outport  Port=2
  wires:
  Cross Product/1 -> Gain3/1
  Constant1/1 -> Gain/1
  Gain/1 -> Reshape/1
  Reshape/1 -> Matrix Multiply/2
  Gain3/1 -> Subtract/1
  Selector/1 -> Gain2/1
  Subtract/1 -> Reshape3/1
  Selector1/1 -> Gain1/1
  Reshape1/1 -> Cross Product/2
  Reshape2/1 -> Cross Product/1
  Saturation1/1 -> a_N_c/1  "a_N_c"
  Saturation2/1 -> a_L_c/1  "a_L_c"
  Reshape3/1 -> Selector/1, Selector1/1
  Switch/1 -> Subtract/2
  Matrix Multiply/1 -> Switch/1
  Constant3/1 -> Switch/2
  Constant2/1 -> Switch/3
  Gain2/1 -> Saturation1/1
  Gain1/1 -> Saturation2/1
  Gain4/1 -> Reshape1/1  "v_BT_B"
  In Bus Element/1 -> Matrix Multiply/1
  In Bus Element1/1 -> Reshape2/1
  In Bus Element2/1 -> Gain4/1

== system Model_6DOF/Guidance system/Optimal Guidance ==
  note: Optimal Guidance
  In Bus Element4 : Inport  PortName=Seeker_Data  Element=s_TB_L
  In Bus Element5 : Inport  PortName=Seeker_Data  Element=v_TB_L
  In Bus Element : Inport  Port=2  PortName=INS_Data  Element=T_BL
  Add : Sum
  Divide : Product  Inputs=*/
  Divide1 : Product  Inputs=*/
  Gain : Gain  Gain=-N
  Gain1 : Gain  Gain=1/g
  Gain2 : Gain  Gain=-1/g
  Matrix Multiply : Product  Multiplication=Matrix(*)
  Reshape3 : Reshape
  Saturation1 : Saturate  UpperLimit=a_N_c_max  LowerLimit=-a_N_c_max
  Saturation2 : Saturate  UpperLimit=a_L_c_max  LowerLimit=-a_L_c_max
  Selector : Selector  InputPortWidth=3  IndexOptions=Index vector (dialog)  Indices=3  OutputSizes=1
  Selector1 : Selector  InputPortWidth=3  IndexOptions=Index vector (dialog)  Indices=2  OutputSizes=1
  Square : Math  Operator=square
  t_go Calculation : Subsystem
  a_N_c : Outport
  a_L_c : Outport  Port=2
  wires:
  Selector/1 -> Gain2/1
  Matrix Multiply/1 -> Reshape3/1
  Selector1/1 -> Gain1/1
  Saturation1/1 -> a_N_c/1  "a_N_c"
  Saturation2/1 -> a_L_c/1  "a_L_c"
  Reshape3/1 -> Selector/1, Selector1/1
  Gain2/1 -> Saturation1/1
  Gain1/1 -> Saturation2/1
  In Bus Element/1 -> Matrix Multiply/1
  In Bus Element4/1 -> Divide/1, t_go Calculation/1(s_TB_L)
  In Bus Element5/1 -> Divide1/1, t_go Calculation/2(v_TB_L)
  t_go Calculation/1(t_go) -> Divide1/2, Square/1
  Square/1 -> Divide/2
  Divide/1 -> Add/1
  Divide1/1 -> Add/2
  Add/1 -> Gain/1
  Gain/1 -> Matrix Multiply/2

== system Model_6DOF/INS/Accel_Triad ==
  f_sp_B : Inport
  Add : Sum
  Add1 : Sum
  Add2 : Sum
  Product : Product  Multiplication=Matrix(*)
  misalignment : Subsystem
  random bias and noise : Subsystem
  scale factor error : Subsystem
  e_f_sp_B : Outport
  f_sp_h_B : Outport  Port=2
  wires:
  misalignment/1(M_a_B) -> Add/2
  scale factor error/1(S_a_B) -> Add/1
  Add/1 -> Product/1
  f_sp_B/1 -> Add2/2, Product/2
  Product/1 -> Add1/2
  random bias and noise/1(e_b_a_B) -> Add1/1
  Add1/1 -> Add2/1, e_f_sp_B/1
  Add2/1 -> f_sp_h_B/1

== system Model_6DOF/INS/Grav_errore ==
  e_s_BE_Lh : Inport
  Constant : Constant  Value=0
  Gain : Gain  Gain=2*g/R_e
  Mux : Mux  Inputs=3
  Reshape : Reshape  OutputDimensionality=Column vector (2-D)
  Selector : Selector  InputPortWidth=3  IndexOptions=Index vector (dialog)  Indices=3  OutputSizes=1
  e_g_Lh : Outport
  wires:
  e_s_BE_Lh/1 -> Selector/1
  Selector/1 -> Gain/1
  Gain/1 -> Mux/3
  Constant/1 -> Mux/2, Mux/1
  Mux/1 -> Reshape/1
  Reshape/1 -> e_g_Lh/1

== system Model_6DOF/INS/Gyro_Triad ==
  f_sp_B : Inport
  omega_BE_B : Inport  Port=2
  Add : Sum
  Add1 : Sum  Inputs=3
  Product : Product  Multiplication=Matrix(*)
  Product1 : Product  Multiplication=Matrix(*)
  imbalance matrix : Subsystem
  misalignment : Subsystem
  random bias and noise : Subsystem
  scale factor error : Subsystem
  e_omega_BE_B : Outport
  wires:
  scale factor error/1(S_g_B) -> Add/1
  misalignment/1(M_g_B) -> Add/2
  Add/1 -> Product/1
  omega_BE_B/1 -> Product/2
  imbalance matrix/1(U_g_B) -> Product1/1
  f_sp_B/1 -> Product1/2
  Product1/1 -> Add1/1
  random bias and noise/1(e_b_g_B) -> Add1/2
  Product/1 -> Add1/3
  Add1/1 -> e_omega_BE_B/1

== system Model_6DOF/INS/Subsystem ==
  s_BE_L : Inport
  Constant : Constant  Value=1/R_e
  Constant1 : Constant  Value=0
  Create 3x3 Matrix : sharedutil/Create 3x3 Matrix  aMode=aMode
  Gain : Gain  Gain=-1
  Product : Product  Inputs=*/
  Product1 : Product
  Selector : Selector  InputPortWidth=3  IndexOptions=Index vector (dialog)  Indices=[1 2]  OutputSizes=1
  Selector2 : Selector  InputPortWidth=3  IndexOptions=Index vector (dialog)  Indices=3  OutputSizes=1
  Sqrt : Sqrt
  Square : Math  Operator=square  SignedPower=on
  Sum of Elements : Sum  Inputs=+
  A : Outport
  wires:
  s_BE_L/1 -> Selector2/1, Selector/1
  Selector/1 -> Square/1
  Square/1 -> Sum of Elements/1
  Sum of Elements/1 -> Sqrt/1
  Selector2/1 -> Product/1
  Sqrt/1 -> Product/2
  Product/1 -> Product1/2  "tan(lambda)"
  Gain/1 -> Product1/1, Create 3x3 Matrix/4
  Constant/1 -> Create 3x3 Matrix/2, Gain/1
  Constant1/1 -> Create 3x3 Matrix/3, Create 3x3 Matrix/6, Create 3x3 Matrix/7, Create 3x3 Matrix/9, Create 3x3 Matrix/5, Create 3x3 Matrix/1
  Product1/1 -> Create 3x3 Matrix/8  "tan(lambda)"
  Create 3x3 Matrix/1 -> A/1

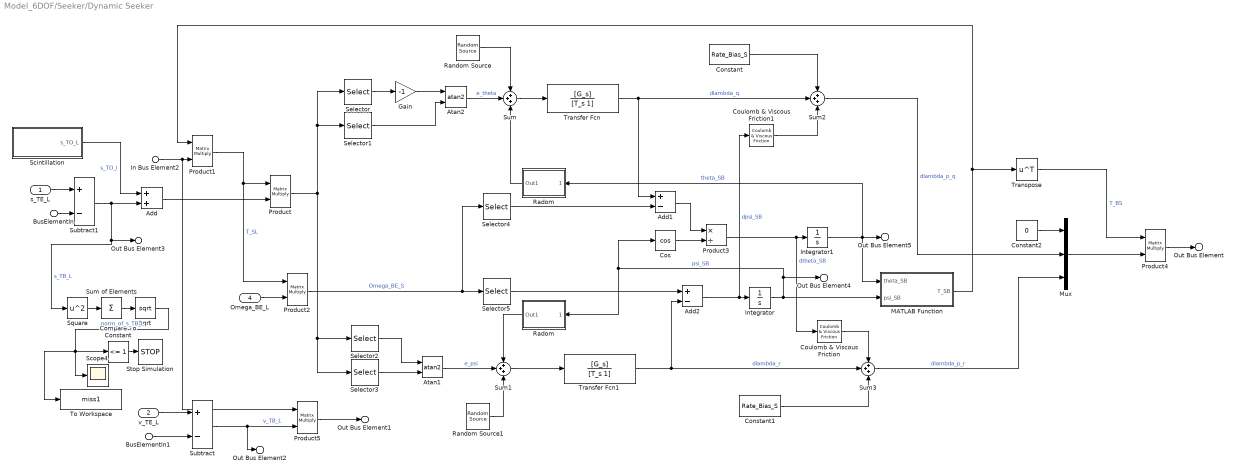
== system Model_6DOF/Seeker/Dynamic Seeker ==
  s_TE_L : Inport
  v_TE_L : Inport  Port=2
  In Bus Element2 : Inport  Port=3  PortName=INS_Data  Element=T_BL
  BusElementIn : Inport  Port=3  PortName=INS_Data  Element=s_BE_L_hat
  BusElementIn1 : Inport  Port=3  PortName=INS_Data  Element=v_BE_L_hat
  Omega_BE_L : Inport  Port=4
  Add : Sum
  Add1 : Sum  Inputs=+-
  Add2 : Sum  Inputs=+-
  Atan1 : Trigonometry  Operator=atan2
  Atan2 : Trigonometry  Operator=atan2
  Compare To Constant : simulink/Logic and Bit Operations/Compare To Constant  relop=<=  const=1  OutDataTypeStr=boolean
  Constant : Constant  Value=Rate_Bias_S
  Constant1 : Constant  Value=Rate_Bias_S
  Constant2 : Constant  Value=0
  Cos : Trigonometry  Operator=cos
  Coulomb & Viscous Friction : simulink/Discontinuities/Coulomb & Viscous Friction  offset=0.01  gain=0
  Coulomb & Viscous Friction1 : simulink/Discontinuities/Coulomb & Viscous Friction  offset=0.01  gain=0
  Gain : Gain  Gain=-1
  Integrator : Integrator  InitialCondition=psi_SB_0
  Integrator1 : Integrator  InitialCondition=theta_SB_0
  MATLAB Function : MATLAB Function  TreatAsAtomicUnit=on
  Mux : Mux  Inputs=3
  Product{,1..2,4..5} (5 alike) : Product  Multiplication=Matrix(*)
  Product3 : Product  Inputs=*/
  Radom : Subsystem
  "Radom " : Subsystem
  Random Source : dspsrcs4/Random Source  SrcType=Uniform  NormMethod=Ziggurat  CltLength=12  MinVal=0  MaxVal=1  MeanVal=0  VarVal=1  RepMode=Not repeatable  rawSeed=1  IsInherit=off  SampMode=Continuous  SampTime=1  SampFrame=1  DataType=Double  OutComplex=Real  OutputFrames=off
  Random Source1 : dspsrcs4/Random Source  SrcType=Uniform  NormMethod=Ziggurat  CltLength=12  MinVal=0  MaxVal=1  MeanVal=0  VarVal=1  RepMode=Not repeatable  rawSeed=1  IsInherit=off  SampMode=Continuous  SampTime=1  SampFrame=1  DataType=Double  OutComplex=Real  OutputFrames=off
  Scintillation : Subsystem
  Scope4 : Scope
  Selector : Selector  InputPortWidth=3  IndexOptions=Index vector (dialog)  Indices=3  OutputSizes=1
  Selector1 : Selector  InputPortWidth=3  IndexOptions=Index vector (dialog)  Indices=1  OutputSizes=1
  Selector2 : Selector  InputPortWidth=3  IndexOptions=Index vector (dialog)  Indices=2  OutputSizes=1
  Selector3 : Selector  InputPortWidth=3  IndexOptions=Index vector (dialog)  Indices=1  OutputSizes=1
  Selector4 : Selector  InputPortWidth=3  IndexOptions=Index vector (dialog)  Indices=2  OutputSizes=1
  Selector5 : Selector  InputPortWidth=3  IndexOptions=Index vector (dialog)  Indices=3  OutputSizes=1
  Sqrt : Sqrt
  Square : Math  Operator=square  SignedPower=on
  Stop Simulation : Stop
  Subtract : Sum  Inputs=+-
  Subtract1 : Sum  Inputs=+-
  Sum{,1..3} (4 alike) : Sum  Inputs=3
  Sum of Elements : Sum  Inputs=+
  To Workspace : ToWorkspace  VariableName=miss1  SampleTime=-1
  Transfer Fcn : TransferFcn  Numerator=[G_s]  Denominator=[T_s 1]
  Transfer Fcn1 : TransferFcn  Numerator=[G_s]  Denominator=[T_s 1]
  Transpose : Math  Operator=transpose
  Out Bus Element : Outport  PortName=Seeker_Data  Element=omega_OE_B
  Out Bus Element1 : Outport  PortName=Seeker_Data  Element=v_TB_B
  Out Bus Element2 : Outport  PortName=Seeker_Data  Element=v_TB_L
  Out Bus Element3 : Outport  PortName=Seeker_Data  Element=s_TB_L
  Out Bus Element4 : Outport  PortName=Seeker_Data  Element=psi_OB
  Out Bus Element5 : Outport  PortName=Seeker_Data  Element=theta_OB
  wires:
  s_TE_L/1 -> Subtract1/1
  Subtract1/1 -> Out Bus Element3/1, Square/1, Add/2  "s_TB_L"
  Scintillation/1(s_TO_L) -> Add/1  "s_TO_l"
  Add/1 -> Product/2
  Product1/1 -> Product/1, Product2/1  "T_SL"
  MATLAB Function/1(T_SB) -> Transpose/1, Product1/1
  In Bus Element2/1 -> Product5/1, Product1/2
  Product/1 -> Selector/1, Selector1/1, Selector3/1, Selector2/1
  Selector/1 -> Gain/1
  Gain/1 -> Atan2/1
  Selector1/1 -> Atan2/2
  Selector2/1 -> Atan1/1
  Selector3/1 -> Atan1/2
  Atan2/1 -> Sum/2  "e_theta"
  Atan1/1 -> Sum1/2  "e_psi"
  Random Source/1 -> Sum/1
  Random Source1/1 -> Sum1/3
  Sum/1 -> Transfer Fcn/1
  Sum1/1 -> Transfer Fcn1/1
  Omega_BE_L/1 -> Product2/2
  Radom/1(Out1) -> Sum/3
  "Radom "/1(Out1) -> Sum1/1
  Transfer Fcn/1 -> Add1/1, Sum2/2  "dlambda_q"
  Selector4/1 -> Add1/2
  Product2/1 -> Selector4/1, Selector5/1  "Omega_BE_S"
  Selector5/1 -> Add2/1
  Transfer Fcn1/1 -> Add2/2, Sum3/2  "dlambda_r"
  Add2/1 -> Coulomb & Viscous Friction1/1, Integrator/1  "dpsi_SB"
  Cos/1 -> Product3/2
  Add1/1 -> Product3/1
  Product3/1 -> Coulomb & Viscous Friction/1, Integrator1/1  "dtheta_SB"
  Integrator1/1 -> Out Bus Element5/1, Radom/1(theta_SB), MATLAB Function/1(theta_SB)  "theta_SB"
  Coulomb & Viscous Friction/1 -> Sum3/1
  Coulomb & Viscous Friction1/1 -> Sum2/3
  Constant/1 -> Sum2/1
  Constant1/1 -> Sum3/3
  Constant2/1 -> Mux/1
  Sum2/1 -> Mux/2  "dlambda_p_q"
  Sum3/1 -> Mux/3  "dlambda_p_r"
  Mux/1 -> Product4/2
  Transpose/1 -> Product4/1  "T_BS"
  v_TE_L/1 -> Subtract/1
  Subtract/1 -> Out Bus Element2/1, Product5/2  "v_TB_L"
  BusElementIn1/1 -> Subtract/2
  Compare To Constant/1 -> Stop Simulation/1
  Sqrt/1 -> To Workspace/1, Scope4/1, Compare To Constant/1  "norm_of_s_TB_L"
  Square/1 -> Sum of Elements/1
  Sum of Elements/1 -> Sqrt/1
  Integrator/1 -> MATLAB Function/2(psi_SB), Out Bus Element4/1, "Radom "/1(psi_SB), Cos/1  "psi_SB"
  BusElementIn/1 -> Subtract1/2
  Product4/1 -> Out Bus Element/1
  Product5/1 -> Out Bus Element1/1

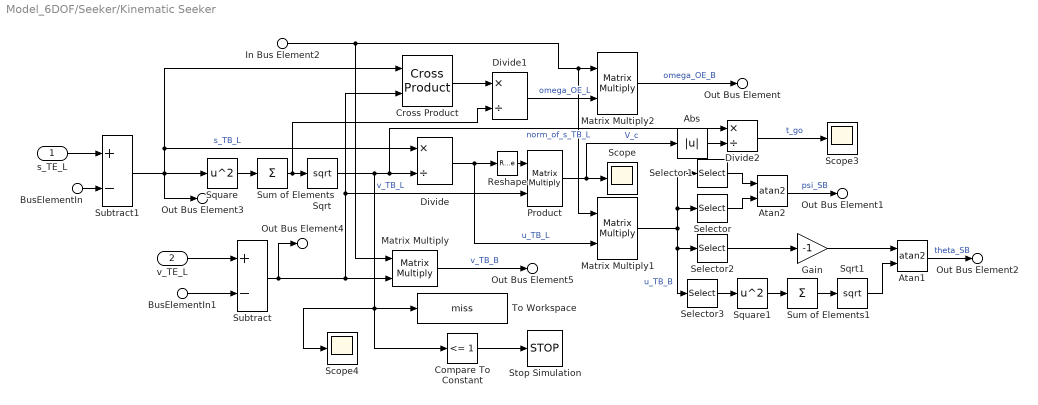
== system Model_6DOF/Seeker/Kinematic Seeker ==
  s_TE_L : Inport
  v_TE_L : Inport  Port=2
  In Bus Element2 : Inport  Port=3  PortName=INS_Data  Element=T_BL
  BusElementIn : Inport  Port=3  PortName=INS_Data  Element=s_BE_L_hat
  BusElementIn1 : Inport  Port=3  PortName=INS_Data  Element=v_BE_L_hat
  Abs : Abs  SaturateOnIntegerOverflow=off
  Atan1 : Trigonometry  Operator=atan2
  Atan2 : Trigonometry  Operator=atan2
  Compare To Constant : simulink/Logic and Bit Operations/Compare To Constant  relop=<=  const=1  OutDataTypeStr=boolean
  Cross Product : matrix_library/Cross Product
  Divide : Product  Inputs=*/
  Divide1 : Product  Inputs=*/
  Divide2 : Product  Inputs=*/
  Gain : Gain  Gain=-1
  Matrix Multiply : Product  Multiplication=Matrix(*)
  Matrix Multiply1 : Product  Multiplication=Matrix(*)
  Matrix Multiply2 : Product  Multiplication=Matrix(*)
  Product : Product  Multiplication=Matrix(*)
  Reshape : Reshape  OutputDimensionality=Row vector (2-D)
  Scope : Scope
  Scope3 : Scope
  Scope4 : Scope
  Selector : Selector  InputPortWidth=3  IndexOptions=Index vector (dialog)  Indices=1  OutputSizes=1
  Selector1 : Selector  InputPortWidth=3  IndexOptions=Index vector (dialog)  Indices=2  OutputSizes=1
  Selector2 : Selector  InputPortWidth=3  IndexOptions=Index vector (dialog)  Indices=3  OutputSizes=1
  Selector3 : Selector  InputPortWidth=3  IndexOptions=Index vector (dialog)  Indices=[1 2]  OutputSizes=1
  Sqrt : Sqrt
  Sqrt1 : Sqrt
  Square : Math  Operator=square  SignedPower=on
  Square1 : Math  Operator=square  SignedPower=on
  Stop Simulation : Stop
  Subtract : Sum  Inputs=+-
  Subtract1 : Sum  Inputs=+-
  Sum of Elements : Sum  Inputs=+
  Sum of Elements1 : Sum  Inputs=+
  To Workspace : ToWorkspace  VariableName=miss  SampleTime=-1
  Out Bus Element : Outport  PortName=Seeker_Data  Element=omega_OE_B
  Out Bus Element1 : Outport  PortName=Seeker_Data  Element=psi_SB
  Out Bus Element2 : Outport  PortName=Seeker_Data  Element=theta_SB
  Out Bus Element3 : Outport  PortName=Seeker_Data  Element=s_TB_L
  Out Bus Element4 : Outport  PortName=Seeker_Data  Element=v_TB_L
  Out Bus Element5 : Outport  PortName=Seeker_Data  Element=v_TB_B
  wires:
  Subtract/1 -> Cross Product/2, Product/2, Matrix Multiply/2, Out Bus Element4/1  "v_TB_L"
  In Bus Element2/1 -> Matrix Multiply1/1, Matrix Multiply2/1, Matrix Multiply/1
  Matrix Multiply/1 -> Out Bus Element5/1  "v_TB_B"
  s_TE_L/1 -> Subtract1/1
  Subtract1/1 -> Out Bus Element3/1, Cross Product/1, Divide/1, Square/1  "s_TB_L"
  Square/1 -> Sum of Elements/1
  Sum of Elements/1 -> Divide1/2, Sqrt/1
  Sqrt/1 -> To Workspace/1, Scope4/1, Compare To Constant/1, Divide2/1, Divide/2  "norm_of_s_TB_L"
  Divide/1 -> Matrix Multiply1/2, Reshape/1  "u_TB_L"
  BusElementIn1/1 -> Subtract/2
  v_TE_L/1 -> Subtract/1
  Cross Product/1 -> Divide1/1
  Divide1/1 -> Matrix Multiply2/2  "omega_OE_L"
  Matrix Multiply2/1 -> Out Bus Element/1  "omega_OE_B"
  Product/1 -> Abs/1, Scope/1  "V_c"
  Matrix Multiply1/1 -> Selector1/1, Selector/1, Selector3/1, Selector2/1  "u_TB_B"
  Selector/1 -> Atan2/2
  Atan2/1 -> Out Bus Element1/1  "psi_SB"
  Selector2/1 -> Gain/1
  Gain/1 -> Atan1/1
  Selector1/1 -> Atan2/1
  Square1/1 -> Sum of Elements1/1
  Selector3/1 -> Square1/1
  Sum of Elements1/1 -> Sqrt1/1
  Sqrt1/1 -> Atan1/2
  Atan1/1 -> Out Bus Element2/1  "theta_SB"
  Abs/1 -> Divide2/2
  Divide2/1 -> Scope3/1  "t_go"
  Reshape/1 -> Product/1
  Compare To Constant/1 -> Stop Simulation/1
  BusElementIn/1 -> Subtract1/2

== system Model_6DOF/Airframe/6DOF Equation of Motion/Rotational Dynamics (kinetics) ==
  Moment : Inport
  p,q,r : Inport  Port=2
  Gyroscopic Moment Due to Rotary Parts : Constant  Value=[l_R;0;0]
  I*w : Product  Multiplication=Matrix(*)
  Moment of Inertia matrix : Constant  Value=I
  Product4 : Product  Inputs=*/  Multiplication=Matrix(*)  SaturateOnIntegerOverflow=on  OutDataTypeStr=Inherit: Same as first input
  "Reshape " : Reshape
  Reshape1 : Reshape  OutputDimensionality=Row vector (2-D)
  Reshape2 : Reshape  OutputDimensionality=Column vector (2-D)
  Reshape3 : Reshape
  Sum1 : Sum  Inputs=-+-  SaturateOnIntegerOverflow=on
  w*(Iw) : sharedutil/3x3 Cross Product  aMode=aMode
  omegadot_body : Outport
  wires:
  Reshape3/1 -> w*(Iw)/2
  I*w/1 -> Reshape3/1
  Reshape2/1 -> w*(Iw)/1, I*w/2
  p,q,r/1 -> Reshape2/1  "p,q,r"
  Moment/1 -> Sum1/2
  Sum1/1 -> Reshape1/1
  w*(Iw)/1 -> Sum1/3
  Product4/1 -> "Reshape "/1
  Moment of Inertia matrix/1 -> Product4/2, I*w/1  "I"
  Reshape1/1 -> Product4/1
  "Reshape "/1 -> omegadot_body/1
  Gyroscopic Moment Due to Rotary Parts/1 -> Sum1/1

== system Model_6DOF/Airframe/6DOF Equation of Motion/Rotational Kinematics ==
  Euler Angles : Inport
  omega_body : Inport  Port=2
  Mux1 : Mux  Inputs=[3 3 3]
  Mux2 : Mux  Inputs=3
  phidot : Fcn  Expr=u[1]+(u[2]*u[4]+u[3]*u[7])*(u[5]/u[8])
  psidot : Fcn  Expr=(u[2]*u[4]+u[3]*u[7])/u[8]
  sincos : Trigonometry  Operator=sincos
  thetadot : Fcn  Expr=u[2]*u[7]-u[3]*u[4]
  Euler Rates : Outport
  wires:
  Euler Angles/1 -> sincos/1  "phi, theta, psi"
  sincos/2 -> Mux1/3
  Mux1/1 -> psidot/1, phidot/1, thetadot/1
  omega_body/1 -> Mux1/1  "p, q, r"
  phidot/1 -> Mux2/1
  psidot/1 -> Mux2/3
  thetadot/1 -> Mux2/2
  sincos/1 -> Mux1/2
  Mux2/1 -> Euler Rates/1

== system Model_6DOF/Airframe/6DOF Equation of Motion/Transitional Dynamics (kinetics) ==
  " F" : Inport
  p,q,r : Inport  Port=2
  V_body : Inport  Port=3
  Constant : Constant  Value=m
  Divide : Product  Inputs=*/
  Sum : Sum  Inputs=+-
  w*Vb : sharedutil/3x3 Cross Product  aMode=aMode
  Vdot_body : Outport
  a_BE_B : Outport  Port=2
  wires:
  p,q,r/1 -> w*Vb/1
  w*Vb/1 -> Sum/2
  Constant/1 -> Divide/2
  Divide/1 -> Sum/1, a_BE_B/1  "F/m"
  Sum/1 -> Vdot_body/1
  V_body/1 -> w*Vb/2
  " F"/1 -> Divide/1

== system Model_6DOF/Airframe/6DOF Equation of Motion/Transitional Kinematics  ==
  V_body : Inport
  Euler Angles : Inport  Port=2
  MatrixMultiply : Product  Multiplication=Matrix(*)
  Reshape : Reshape
  Reshape3 : Reshape  OutputDimensionality=Column vector (2-D)
  Rotation Angles to Direction Cosine Matrix : sharedtransform/Rotation Angles to Direction Cosine Matrix  rotationOrder=ZYX  aMode=aMode
  Selector : Selector  InputPortWidth=3  IndexOptions=Index vector (dialog)  Indices=[3 2 1]  OutputSizes=1
  Transpose : Math  Operator=transpose
  V_earth : Outport
  wires:
  Reshape/1 -> V_earth/1
  MatrixMultiply/1 -> Reshape/1
  Reshape3/1 -> MatrixMultiply/2
  V_body/1 -> Reshape3/1
  Rotation Angles to Direction Cosine Matrix/1 -> Transpose/1
  Transpose/1 -> MatrixMultiply/1
  Selector/1 -> Rotation Angles to Direction Cosine Matrix/1
  Euler Angles/1 -> Selector/1

== system Model_6DOF/Airframe/Forces and Moments (in Body)/Aerodynamics Forces & Moments ==
  note: Control Surface Deflections
  v : Inport
  alpha : Inport  Port=2
  beta : Inport  Port=3
  CSD : Inport  Port=4
  rho : Inport  Port=5
  omega_BE_B : Inport  Port=6
  Aerodynamics Forces (body) : Subsystem
  Aerodynamics Moments (body) : Subsystem
  Demux : Demux  Outputs=3
  F_A_B : Outport
  M_A_B : Outport  Port=2
  wires:
  rho/1 -> Aerodynamics Moments (body)/5(rho), Aerodynamics Forces (body)/8(rho)
  v/1 -> Aerodynamics Forces (body)/2(v), Aerodynamics Moments (body)/2(v)
  Demux/1 -> Aerodynamics Moments (body)/6(de), Aerodynamics Forces (body)/5(de)  "de"
  Demux/2 -> Aerodynamics Forces (body)/6(da), Aerodynamics Moments (body)/7(da)  "da"
  Aerodynamics Forces (body)/1(F_A_B) -> F_A_B/1
  alpha/1 -> Aerodynamics Moments (body)/3(alpha), Aerodynamics Forces (body)/3(alpha)
  beta/1 -> Aerodynamics Moments (body)/4(beta), Aerodynamics Forces (body)/4(beta)
  Demux/3 -> Aerodynamics Moments (body)/8(dr), Aerodynamics Forces (body)/7(dr)  "dr"
  Aerodynamics Moments (body)/1(M_A_B) -> M_A_B/1
  CSD/1 -> Demux/1
  omega_BE_B/1 -> Aerodynamics Moments (body)/1(omega_BE_B), Aerodynamics Forces (body)/1(omega_BE_B)
